simulink model "ANC"  (R2023b)
settings: Solver=VariableStepAuto  StartTime=0.0  StopTime=1000  RelTol=1e-3
libraries: dspadpt3 x1
settings Model: Creator=q  LastModifiedBy=q

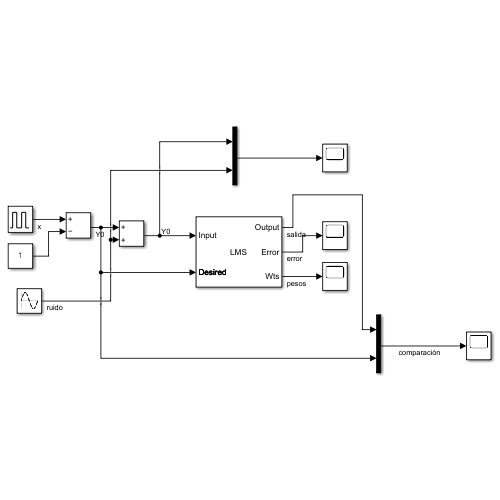
[thumbnail: Simulink's stored preview of the top-level diagram]
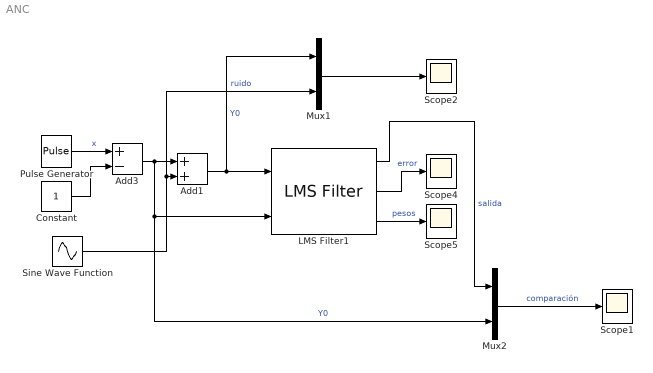
== system ANC ==
  Add1 : Sum
  Add3 : Sum  Inputs=+-
  Constant : Constant
  LMS Filter1 : dspadpt3/LMS Filter  Algo=LMS  L=100  stepflag=Dialog  mu=0.01  leakage=1.0  ic=0  Adapt=off  resetflag=None  weights=on  addnparflag=off  roundingMode=Floor  overflowMode=off
  Mux1 : Mux  Inputs=2
  Mux2 : Mux  Inputs=2
  Pulse Generator : DiscretePulseGenerator  PulseType=Time based  Amplitude=2  Period=0.1  PulseWidth=50
  Scope{1..2,4..5} (4 alike) : Scope
  Sine Wave Function : Sin  Frequency=60  SampleTime=0
  wires:
  Mux1/1 -> Scope2/1
  Add1/1 -> Mux1/1, LMS Filter1/1  "Y0"
  Pulse Generator/1 -> Add3/1  "x"
  Constant/1 -> Add3/2
  Add3/1 -> LMS Filter1/2, Mux2/2, Add1/1  "Y0"
  Sine Wave Function/1 -> Mux1/2, Add1/2  "ruido"
  LMS Filter1/1 -> Mux2/1  "salida"
  LMS Filter1/2 -> Scope4/1  "error"
  LMS Filter1/3 -> Scope5/1  "pesos"
  Mux2/1 -> Scope1/1  "comparación"
